simulink model "HESS_Passive_structure"  (R2014a)
settings: Solver=ode45  StartTime=0.0  StopTime=1377  FixedStep=0.001  MaxStep=0.005  RelTol=1e-3
undefined symbols (not defined in the file or in its folder): Ion, Lithium
libraries: powerlib x8, electricdrivelib x1
settings Model: Creator=Administrator  LastModifiedBy=Administrator
settings SolverCC: AlgebraicLoopSolver=LineSearch
settings DataIOCC: SignalLoggingSaveFormat=ModelDataLogs
settings OptimizationCC: ExpressionDepthLimit=2147483647
settings DebuggingCC: UnderspecifiedInitializationDetection=Classic  FcnCallInpInsideContextMsg=UseLocalSettings  StateNameClashWarn=warning
settings GRTTargetCC: CombineOutputUpdateFcns=off  GRTInterface=on

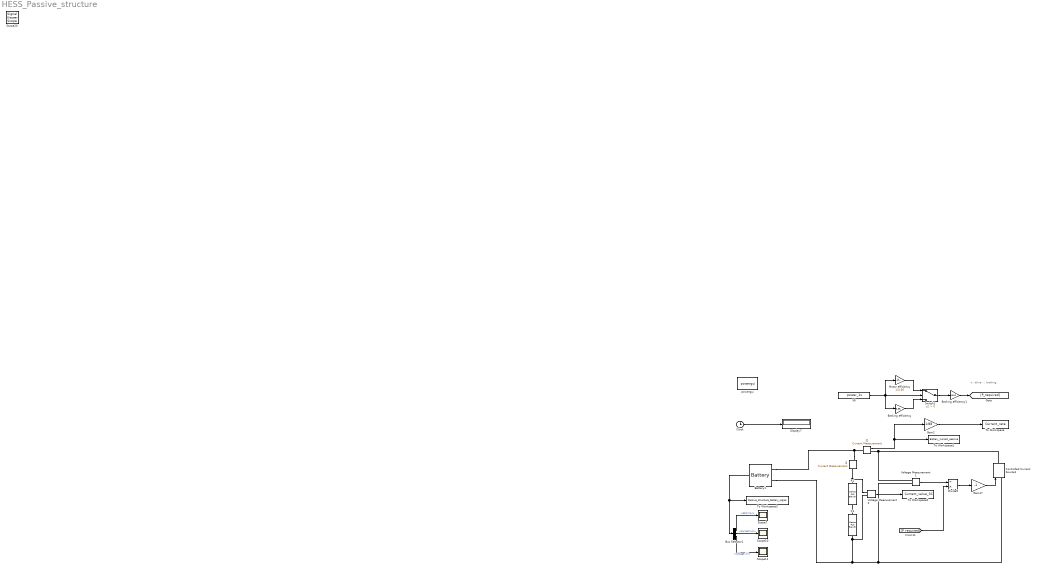
== system HESS_Passive_structure ==
  note: +: drive
      | - : braking
  Battery1 : electricdrivelib/Extra Sources/Battery  BatType=Lithium-Ion  ShowDetailedParameters=on  NomV=259.25  NomQ=88  SOC=90  PresetModel=on  MaxQ=88  FullV=301.7637  Dis_rate=38.2609  R=0.02946  Normal_OP=79.5826  expZone="[280.09      4.323478]"  Dis_Char=off  current=[1.5 3]  Units=Ampere-hour  Batt_Tr=30
  Braking efficiency : Gain  Gain=0.35
  Braking efficiency1 : Gain  Gain=1000
  Bus Selector1 : BusSelector  OutputSignals=SOC (%),Current (A),Voltage (V)
  C1 : powerlib/Elements/Series RLC Branch  LConnTagsString=__new0  RConnTagsString=__new0  BranchType=C  Resistance=1  Inductance=1e-3  SetiL0=off  InitialCurrent=0  Capacitance=15.1  Setx0=on  InitialVoltage=356  Measurements=Branch voltage
  Clock : Clock
  Controlled Current Source1 : powerlib/Electrical Sources/Controlled Current Source  Initialize=on  Source_Type=AC  Amplitude=0  Phase=0  Frequency=0  Measurements=None
  Display7 : Display
  Divide5 : Product  Inputs=/*
  Gain17 : Gain  Gain=-1
  Gain2 : Gain  Gain=1/88
  I1 : powerlib/Measurements/Current Measurement  PhasorSimulation=off  OutputType=Complex  PSBequivalent=0
  I2 : powerlib/Measurements/Current Measurement  PhasorSimulation=off  OutputType=Complex  PSBequivalent=0
  Motor efficiency : Gain  Gain=1/0.95
  R1 : powerlib/Elements/Series RLC Branch  LConnTagsString=__new0  RConnTagsString=__new0  BranchType=R  Resistance=0.0462  Inductance=1e-3  SetiL0=off  InitialCurrent=0  Capacitance=1e-6  Setx0=off  InitialVoltage=0  Measurements=None
  Scope10 : Scope
      settings: SaveName=ScopeData9
  Scope11 : Scope
      settings: YMin=409  YMax=419.5  SaveName=ScopeData13
  Scope7 : Scope
      settings: YMin=92  YMax=95.25  SaveName=ScopeData14
  Switch1 : Switch  Criteria=u2 > Threshold
  To Workspace : ToWorkspace  VariableName=Current_rate  SampleTime=-1
  To Workspace1 : ToWorkspace  VariableName=Battery_current_passive  SampleTime=-1
  To Workspace2 : ToWorkspace  VariableName=Current_value_SC  SampleTime=-1
  To Workspace3 : ToWorkspace  VariableName=Passive_structure_battery_signal  SampleTime=-1
  V6 : FromWorkspace  VariableName=power_1s  SampleTime=1
  Voltage Measurement1 : powerlib/Measurements/Voltage Measurement  PhasorSimulation=off  OutputType=Complex  PSBequivalent=0
  Voltage Measurement2 : powerlib/Measurements/Voltage Measurement  PhasorSimulation=off  OutputType=Complex  PSBequivalent=0
  powergui : powerlib/powergui  Priority=1  SimulationMode=Discrete  SolverType=Tustin  SampleTime=1  frequency=60  SPID=off  DisableSnubberDevices=off  DisableRonSwitches=off  DisableVfSwitches=off  SwTol=0  Interpol=off  DisplayEquations=off  Ts=0  methode=off  frequencyindice=0  Pbase=100e6  ErrMax=1e-4  Iterations=50  UnitsV=kV  UnitsW=MW  FunctionMessages=off  echomessages=off  HookPort=off  EnableUseOfTLC=off  x0status=blocks  RestoreLinks=warning  ResistiveCurrentMeasurement=off  Frange=[0:2:500]  Ylog=off  Xlog=on  ShowGrid=off  save=off  variable=ZData  structure=0  ZoomFFT=off  StartTime=0.0  cycles=1  DisplayStyle=1  fundamental=60  FreqAxis=off  MaxFrequency=1000  frequencyindicesteady=1  RmsSteady=1  display=off
  Scope20 : SignalViewerScope  IOType=viewer  RefreshTime=0.035000
  wires:
  Battery1/1 -> To Workspace3/1, Bus Selector1/1
  Bus Selector1/1 -> Scope7/1  "<SOC (%)>"
  Bus Selector1/2 -> Scope10/1  "<Current (A)>"
  Bus Selector1/3 -> Scope11/1  "<Voltage (V)>"
  Divide5/1 -> Gain17/1
  Clock/1 -> Display7/1
  Gain17/1 -> Controlled Current Source1/1
  Voltage Measurement1/1 -> Divide5/1
  I2/1 -> To Workspace1/1, Gain2/1
  Gain2/1 -> To Workspace/1
  [P_required] -> Divide5/2
  Voltage Measurement2/1 -> To Workspace2/1
  V6/1 -> Motor efficiency/1, Braking efficiency/1, Switch1/2
  Motor efficiency/1 -> Switch1/1
  Braking efficiency/1 -> Switch1/3
  Switch1/1 -> Braking efficiency1/1
  Braking efficiency1/1 -> [P_required]
  connections:
  I1/RConn1 -- Battery1/LConn1 -- I2/LConn1
  Controlled Current Source1/RConn1 -- Voltage Measurement1/LConn1 -- I2/RConn1
  C1/RConn1 -- Voltage Measurement2/LConn2 -- Battery1/LConn2 -- Voltage Measurement1/LConn2 -- Controlled Current Source1/LConn1
  Voltage Measurement2/LConn1 -- I1/LConn1 -- R1/LConn1
  R1/RConn1 -- C1/LConn1
